simulink subsystem "gravity_simple"  (R2020a)
settings: Solver=VariableStepAuto  StartTime=0.0  StopTime=10.0  RelTol=1e-3
settings Model: Creator=Philip  LastModifiedBy=Philip

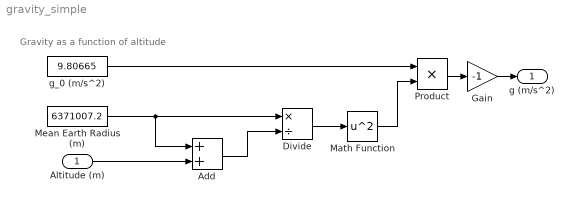
== system gravity_simple ==
  note: Gravity as a function of altitude
  Altitude (m) : Inport
  Add : Sum
  Divide : Product  Inputs=*/
  Gain : Gain  Gain=-1
  Math Function : Math  Operator=square  SaturateOnIntegerOverflow=on
  Mean Earth Radius (m) : Constant  Value=6371007.2
  Product : Product
  g_0 (m/s^2) : Constant  Value=9.80665
  g (m/s^2) : Outport
  wires:
  Gain/1 -> g (m/s^2)/1
  Product/1 -> Gain/1
  Math Function/1 -> Product/2
  g_0 (m/s^2)/1 -> Product/1
  Divide/1 -> Math Function/1
  Add/1 -> Divide/2
  Altitude (m)/1 -> Add/2
  Mean Earth Radius (m)/1 -> Divide/1, Add/1
